simulink model "ProjectOverview"  (R2016a)
settings: Solver=VariableStepAuto  StartTime=0.0  StopTime=1  RelTol=1e-3
libraries: fl_lib x36, elec_lib x17, nesl_utility x6
settings Model: Creator=Peter  LastModifiedBy=Peter

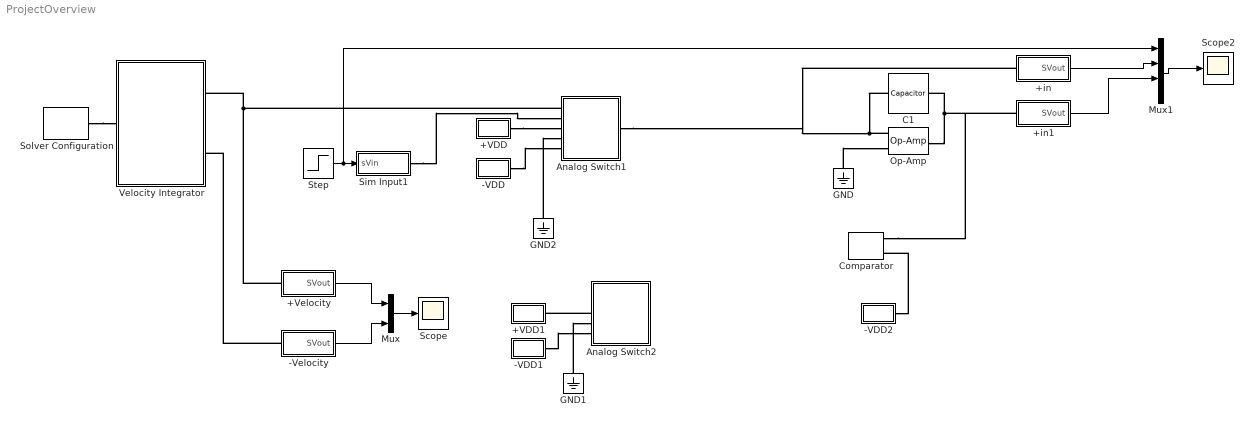
== system ProjectOverview ==
  +VDD : Subsystem
  +VDD1 : Subsystem
  +Velocity : Subsystem
  +in : Subsystem
  +in1 : Subsystem
  -VDD : Subsystem
  -VDD1 : Subsystem
  -VDD2 : Subsystem
  -Velocity : Subsystem
  Analog Switch1 : Subsystem
  Analog Switch2 : Subsystem
  C1 : fl_lib/Electrical/Electrical Elements/Capacitor  c=1e-6 F  r=1e-6 Ohm  g=0 1/Ohm  i_specify=off  i_priority=None  i=0 A  v_specify=off  v_priority=None  v=0 V  vc_specify=off  vc_priority=High  vc=0 V
  Comparator : elec_lib/Integrated Circuits/Comparator  V_OS=5 mV  V_OL=-14.3 V  V_OH=14.3 V  C_IN=0 pF  R_OUT=50 Ohm  Delay=0 s
  GND : fl_lib/Electrical/Electrical Elements/Electrical Reference
  GND1 : fl_lib/Electrical/Electrical Elements/Electrical Reference
  GND2 : fl_lib/Electrical/Electrical Elements/Electrical Reference
  Mux : Mux  Inputs=2
  Mux1 : Mux
  Op-Amp : fl_lib/Electrical/Electrical Elements/Op-Amp  outI_specify=off  outI_priority=None  outI=0 A
  Scope : Scope
  Scope2 : Scope
  Sim Input1 : Subsystem
  Solver Configuration : nesl_utility/Solver Configuration  PhysicalDomain=network_engine_domain  SubClassName=solver  LeftPortType=input  RightPortType=generic  Accelerate=off  Tones=[]  Harmonics=[]  SimulateNoise=off  Profile=off  UseLocalSampling=off  EnableSwitchedLinearOptims=on  FrequencyDomain=off  UseCCode=off  RelTol=0.001  AbsTol=1e-06  MinStep=1e-09  ToWorkspace=off  RevertToSquareIcSolve=off  NumHomotopyIterations=100  PhasorMode=off  PhasorModeNumHarmonics=1  OverrideAbsTol=off  DoDC=off  ResidualTolerance=1e-09  UseLocalSolver=off  LocalSolverChoice=NE_BACKWARD_EULER_ADVANCER  LocalSolverSampleTime=0.001  DoFixedCost=off  MaxNonlinIter=3  MaxModeIter=2  LinearAlgebra=Sparse  DelaysMemoryBudget=1024  AutomaticFiltering=on  FilteringTimeConstant=0.001
  Step : Step  Time=.5  Before=-10  After=10  SampleTime=0
  Velocity Integrator : Subsystem
  wires:
  +Velocity/1(SVout) -> Mux/1
  -Velocity/1(SVout) -> Mux/2
  Mux/1 -> Scope/1
  Mux1/1 -> Scope2/1
  +in/1(SVout) -> Mux1/2
  +in1/1(SVout) -> Mux1/3
  Step/1 -> Mux1/1, Sim Input1/1(sVin)
  connections:
  Solver Configuration/RConn1 -- Velocity Integrator/LConn1
  GND/LConn1 -- Op-Amp/LConn1
  Op-Amp/RConn1 -- Comparator/LConn2 -- +in1/LConn1 -- C1/RConn1
  +Velocity/LConn1 -- Analog Switch1/LConn1 -- Velocity Integrator/RConn1
  -Velocity/LConn1 -- Velocity Integrator/RConn2
  Op-Amp/LConn2 -- Analog Switch1/RConn1 -- +in/LConn1 -- C1/LConn1
  +VDD/RConn1 -- Analog Switch1/LConn3
  -VDD/RConn1 -- Analog Switch1/LConn5
  GND2/LConn1 -- Analog Switch1/LConn4
  Sim Input1/RConn1 -- Analog Switch1/LConn2
  Analog Switch2/LConn3 -- +VDD1/RConn1
  -VDD1/RConn1 -- Analog Switch2/LConn5
  GND1/LConn1 -- Analog Switch2/LConn4
  -VDD2/RConn1 -- Comparator/LConn1

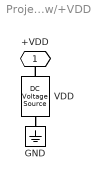
== system ProjectOverview/+VDD ==
  GND : fl_lib/Electrical/Electrical Elements/Electrical Reference
  VDD : fl_lib/Electrical/Electrical Sources/DC Voltage Source  v0=14.3 V
  +VDD : PMIOPort  Port=1  Side=Right
  connections:
  VDD/LConn1 -- +VDD/RConn1
  VDD/RConn1 -- GND/LConn1

== system ProjectOverview/+VDD1 ==
  GND : fl_lib/Electrical/Electrical Elements/Electrical Reference
  VDD : fl_lib/Electrical/Electrical Sources/DC Voltage Source  v0=14.3 V
  +VDD : PMIOPort  Port=1  Side=Right
  connections:
  VDD/LConn1 -- +VDD/RConn1
  VDD/RConn1 -- GND/LConn1

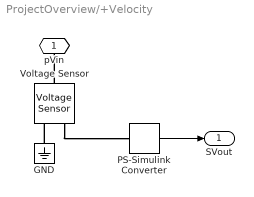
== system ProjectOverview/+Velocity ==
  GND : fl_lib/Electrical/Electrical Elements/Electrical Reference
  PS-Simulink Converter : nesl_utility/PS-Simulink Converter  PhysicalDomain=network_engine_domain  SubClassName=ps_output  LeftPortType=input  RightPortType=output  PseudoPeriodic=off  Frequencies=[]  Unit=V  AffineConversion=off
  Voltage Sensor : fl_lib/Electrical/Electrical Sensors/Voltage Sensor
  pVin : PMIOPort  Port=1  Side=Left
  SVout : Outport
  wires:
  PS-Simulink Converter/1 -> SVout/1
  connections:
  GND/LConn1 -- Voltage Sensor/RConn2
  Voltage Sensor/LConn1 -- pVin/RConn1
  Voltage Sensor/RConn1 -- PS-Simulink Converter/LConn1

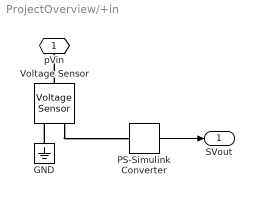
== system ProjectOverview/+in ==
  GND : fl_lib/Electrical/Electrical Elements/Electrical Reference
  PS-Simulink Converter : nesl_utility/PS-Simulink Converter  PhysicalDomain=network_engine_domain  SubClassName=ps_output  LeftPortType=input  RightPortType=output  PseudoPeriodic=off  Frequencies=[]  Unit=V  AffineConversion=off
  Voltage Sensor : fl_lib/Electrical/Electrical Sensors/Voltage Sensor
  pVin : PMIOPort  Port=1  Side=Left
  SVout : Outport
  wires:
  PS-Simulink Converter/1 -> SVout/1
  connections:
  GND/LConn1 -- Voltage Sensor/RConn2
  Voltage Sensor/LConn1 -- pVin/RConn1
  Voltage Sensor/RConn1 -- PS-Simulink Converter/LConn1

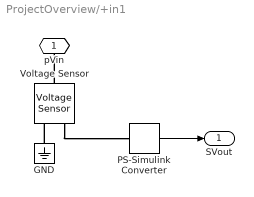
== system ProjectOverview/+in1 ==
  GND : fl_lib/Electrical/Electrical Elements/Electrical Reference
  PS-Simulink Converter : nesl_utility/PS-Simulink Converter  PhysicalDomain=network_engine_domain  SubClassName=ps_output  LeftPortType=input  RightPortType=output  PseudoPeriodic=off  Frequencies=[]  Unit=V  AffineConversion=off
  Voltage Sensor : fl_lib/Electrical/Electrical Sensors/Voltage Sensor
  pVin : PMIOPort  Port=1  Side=Left
  SVout : Outport
  wires:
  PS-Simulink Converter/1 -> SVout/1
  connections:
  GND/LConn1 -- Voltage Sensor/RConn2
  Voltage Sensor/LConn1 -- pVin/RConn1
  Voltage Sensor/RConn1 -- PS-Simulink Converter/LConn1

== system ProjectOverview/-VDD ==
  GND : fl_lib/Electrical/Electrical Elements/Electrical Reference
  VDD : fl_lib/Electrical/Electrical Sources/DC Voltage Source  v0=14.3 V
  -VDD : PMIOPort  Port=1  Side=Right
  connections:
  VDD/RConn1 -- -VDD/RConn1
  GND/LConn1 -- VDD/LConn1

== system ProjectOverview/-VDD1 ==
  GND : fl_lib/Electrical/Electrical Elements/Electrical Reference
  VDD : fl_lib/Electrical/Electrical Sources/DC Voltage Source  v0=14.3 V
  -VDD : PMIOPort  Port=1  Side=Right
  connections:
  VDD/RConn1 -- -VDD/RConn1
  GND/LConn1 -- VDD/LConn1

== system ProjectOverview/-VDD2 ==
  GND : fl_lib/Electrical/Electrical Elements/Electrical Reference
  VDD : fl_lib/Electrical/Electrical Sources/DC Voltage Source  v0=14.3 V
  -VDD : PMIOPort  Port=1  Side=Right
  connections:
  VDD/RConn1 -- -VDD/RConn1
  GND/LConn1 -- VDD/LConn1

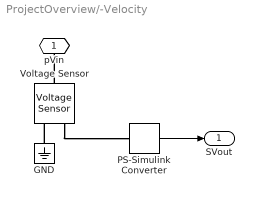
== system ProjectOverview/-Velocity ==
  GND : fl_lib/Electrical/Electrical Elements/Electrical Reference
  PS-Simulink Converter : nesl_utility/PS-Simulink Converter  PhysicalDomain=network_engine_domain  SubClassName=ps_output  LeftPortType=input  RightPortType=output  PseudoPeriodic=off  Frequencies=[]  Unit=V  AffineConversion=off
  Voltage Sensor : fl_lib/Electrical/Electrical Sensors/Voltage Sensor
  pVin : PMIOPort  Port=1  Side=Left
  SVout : Outport
  wires:
  PS-Simulink Converter/1 -> SVout/1
  connections:
  GND/LConn1 -- Voltage Sensor/RConn2
  Voltage Sensor/LConn1 -- pVin/RConn1
  Voltage Sensor/RConn1 -- PS-Simulink Converter/LConn1

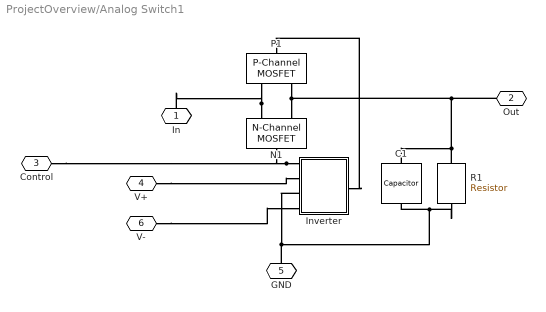
== system ProjectOverview/Analog Switch1 ==
  C1 : fl_lib/Electrical/Electrical Elements/Capacitor  c=1e-6 F  r=1e-6 Ohm  g=0 1/Ohm  i_specify=off  i_priority=None  i=0 A  v_specify=off  v_priority=None  v=0 V  vc_specify=off  vc_priority=High  vc=0 V
  Inverter : Subsystem
  N1 : elec_lib/Semiconductor Devices/N-Channel MOSFET  parameterization=1  prmDatasheet=1  prmEquCoeff=1  Beta=5 A/V^2  Rds=0.025 Ohm  Id=6 A  Vgs=10 V  Vth=1.7 V  lam=0 1/V  Tmeas=25 degC  RS=1e-4 Ohm  RD=0.01 Ohm  C_param=1  C_GS=270 pF  C_GD=80 pF  C_DS=0 pF  C_iss=350 pF  C_rss=80 pF  C_oss=0 pF  C_GS_vec=[ 270 300 290 280 295 255 ] pF  C_GD_vec=[ 450 400 300 190 95 55 ] pF  C_DS_vec=[ 450 410 390 230 175 115 ] pF  C_iss_vec=[ 720 700 590 470 390 310 ] pF  C_rss_vec=[ 450 400 300 190 95 55 ] pF  C_oss_vec=[ 900 810 690 420 270 170 ] pF  C_Vds_vec=[ 0.1 0.3 1 3 10 30 ] V  charge_linearity_param=1  C_OX=200 pF  V_C_OX=-0.5 V  dVth_dT=-6 mV/K  Rds_T2=0.037 Ohm  Tmeas2=125 degC  BEXDatasheet=-1.5  BEXEquCoeff=-1.5  TdeviceDatasheet=25 degC  TdeviceEquCoeff=25 degC  Rth=[ 0 10 ] K/W  thermal_mass_parameterization=1  thermal_mass=[ 0 1 ] J/K  thermal_time_constant=[ 0 10 ] s  thermal_mass_initial_temperatures=[ 25 25 ] degC
  P1 : elec_lib/Semiconductor Devices/P-Channel MOSFET  parameterization=1  prmDatasheet=1  prmEquCoeff=1  Beta=2 A/V^2  Rds=0.167 Ohm  Id=-2.5 A  Vgs=-4.5 V  Vth=-1.4 V  lam=0 1/V  Tmeas=25 degC  RS=1e-4 Ohm  RD=0.01 Ohm  C_param=1  C_GS=158 pF  C_GD=24 pF  C_DS=0 pF  C_iss=182 pF  C_rss=24 pF  C_oss=0 pF  C_GS_vec=[ 150 150 150 150 150 150 ] pF  C_GD_vec=[ 75 60 50 35 25 20 ] pF  C_DS_vec=[ 105 100 75 45 35 25 ] pF  C_iss_vec=[ 225 210 200 185 175 170 ] pF  C_rss_vec=[ 75 60 50 35 25 20 ] pF  C_oss_vec=[ 180 160 125 80 60 45 ] pF  C_Vsd_vec=[ 0.1 0.3 1 3 10 30 ] V  charge_linearity_param=1  C_OX=200 pF  V_C_OX=0.5 V  dVth_dT=2 mV/K  Rds_T2=0.25 Ohm  Tmeas2=125 degC  BEXDatasheet=-1.5  BEXEquCoeff=-1.5  TdeviceDatasheet=25 degC  TdeviceEquCoeff=25 degC  Rth=[ 0 10 ] K/W  thermal_mass_parameterization=1  thermal_mass=[ 0 1 ] J/K  thermal_time_constant=[ 0 10 ] s  thermal_mass_initial_temperatures=[ 25 25 ] degC
  R1 : elec_lib/Passive Devices/Resistor  R=100e3 Ohm  R_tol=5  enable_R_tol=0  tol_distribution=1  nSigma=4  enable_operating_limits=0  operating_limit_action=2  max_working_voltage=100 V  power_rating=1 W  enable_faults=0  fault_action=1  R_faulted=Inf Ohm  enable_temporal_fault=0  t_fault=1 s  enable_behavioral_fault=0  max_permissible_current=1 A  t_fail_on_current=1 s  noise_mode=0  sample_time=0.001 s  repeatability=1  auto_seed=1099607551  user_seed=0  Tdevice=25 degC  alpha=0.00393 1/K  Tmeas=25 degC  thermal_mass=100 J/K  initial_temperature=25 degC  power_derating_T1=70 degC  power_derating_T2=155 degC  operating_temperature_range_vec=[ -50 150 ] degC
  In : PMIOPort  Port=1  Side=Left
  Out : PMIOPort  Port=2  Side=Right
  Control : PMIOPort  Port=3  Side=Left
  V+ : PMIOPort  Port=4  Side=Left
  GND : PMIOPort  Port=5  Side=Left
  V- : PMIOPort  Port=6  Side=Left
  connections:
  GND/RConn1 -- C1/RConn1 -- R1/RConn1 -- Inverter/LConn3
  Inverter/RConn1 -- P1/LConn1
  Inverter/LConn1 -- N1/LConn1 -- Control/RConn1
  C1/LConn1 -- R1/LConn1 -- N1/RConn1 -- P1/RConn2 -- Out/RConn1
  N1/RConn2 -- P1/RConn1 -- In/RConn1
  V+/RConn1 -- Inverter/LConn2
  V-/RConn1 -- Inverter/LConn4

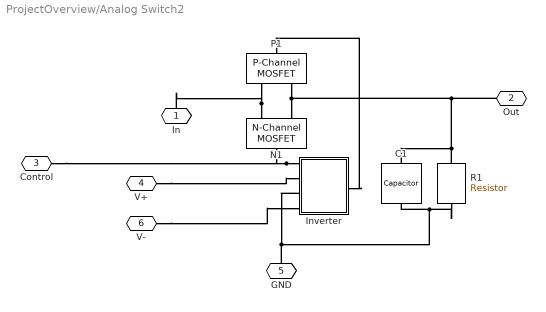
== system ProjectOverview/Analog Switch2 ==
  C1 : fl_lib/Electrical/Electrical Elements/Capacitor  c=1e-6 F  r=1e-6 Ohm  g=0 1/Ohm  i_specify=off  i_priority=None  i=0 A  v_specify=off  v_priority=None  v=0 V  vc_specify=off  vc_priority=High  vc=0 V
  Inverter : Subsystem
  N1 : elec_lib/Semiconductor Devices/N-Channel MOSFET  parameterization=1  prmDatasheet=1  prmEquCoeff=1  Beta=5 A/V^2  Rds=0.025 Ohm  Id=6 A  Vgs=10 V  Vth=1.7 V  lam=0 1/V  Tmeas=25 degC  RS=1e-4 Ohm  RD=0.01 Ohm  C_param=1  C_GS=270 pF  C_GD=80 pF  C_DS=0 pF  C_iss=350 pF  C_rss=80 pF  C_oss=0 pF  C_GS_vec=[ 270 300 290 280 295 255 ] pF  C_GD_vec=[ 450 400 300 190 95 55 ] pF  C_DS_vec=[ 450 410 390 230 175 115 ] pF  C_iss_vec=[ 720 700 590 470 390 310 ] pF  C_rss_vec=[ 450 400 300 190 95 55 ] pF  C_oss_vec=[ 900 810 690 420 270 170 ] pF  C_Vds_vec=[ 0.1 0.3 1 3 10 30 ] V  charge_linearity_param=1  C_OX=200 pF  V_C_OX=-0.5 V  dVth_dT=-6 mV/K  Rds_T2=0.037 Ohm  Tmeas2=125 degC  BEXDatasheet=-1.5  BEXEquCoeff=-1.5  TdeviceDatasheet=25 degC  TdeviceEquCoeff=25 degC  Rth=[ 0 10 ] K/W  thermal_mass_parameterization=1  thermal_mass=[ 0 1 ] J/K  thermal_time_constant=[ 0 10 ] s  thermal_mass_initial_temperatures=[ 25 25 ] degC
  P1 : elec_lib/Semiconductor Devices/P-Channel MOSFET  parameterization=1  prmDatasheet=1  prmEquCoeff=1  Beta=2 A/V^2  Rds=0.167 Ohm  Id=-2.5 A  Vgs=-4.5 V  Vth=-1.4 V  lam=0 1/V  Tmeas=25 degC  RS=1e-4 Ohm  RD=0.01 Ohm  C_param=1  C_GS=158 pF  C_GD=24 pF  C_DS=0 pF  C_iss=182 pF  C_rss=24 pF  C_oss=0 pF  C_GS_vec=[ 150 150 150 150 150 150 ] pF  C_GD_vec=[ 75 60 50 35 25 20 ] pF  C_DS_vec=[ 105 100 75 45 35 25 ] pF  C_iss_vec=[ 225 210 200 185 175 170 ] pF  C_rss_vec=[ 75 60 50 35 25 20 ] pF  C_oss_vec=[ 180 160 125 80 60 45 ] pF  C_Vsd_vec=[ 0.1 0.3 1 3 10 30 ] V  charge_linearity_param=1  C_OX=200 pF  V_C_OX=0.5 V  dVth_dT=2 mV/K  Rds_T2=0.25 Ohm  Tmeas2=125 degC  BEXDatasheet=-1.5  BEXEquCoeff=-1.5  TdeviceDatasheet=25 degC  TdeviceEquCoeff=25 degC  Rth=[ 0 10 ] K/W  thermal_mass_parameterization=1  thermal_mass=[ 0 1 ] J/K  thermal_time_constant=[ 0 10 ] s  thermal_mass_initial_temperatures=[ 25 25 ] degC
  R1 : elec_lib/Passive Devices/Resistor  R=100e3 Ohm  R_tol=5  enable_R_tol=0  tol_distribution=1  nSigma=4  enable_operating_limits=0  operating_limit_action=2  max_working_voltage=100 V  power_rating=1 W  enable_faults=0  fault_action=1  R_faulted=Inf Ohm  enable_temporal_fault=0  t_fault=1 s  enable_behavioral_fault=0  max_permissible_current=1 A  t_fail_on_current=1 s  noise_mode=0  sample_time=0.001 s  repeatability=1  auto_seed=2017132988  user_seed=0  Tdevice=25 degC  alpha=0.00393 1/K  Tmeas=25 degC  thermal_mass=100 J/K  initial_temperature=25 degC  power_derating_T1=70 degC  power_derating_T2=155 degC  operating_temperature_range_vec=[ -50 150 ] degC
  In : PMIOPort  Port=1  Side=Left
  Out : PMIOPort  Port=2  Side=Right
  Control : PMIOPort  Port=3  Side=Left
  V+ : PMIOPort  Port=4  Side=Left
  GND : PMIOPort  Port=5  Side=Left
  V- : PMIOPort  Port=6  Side=Left
  connections:
  GND/RConn1 -- C1/RConn1 -- R1/RConn1 -- Inverter/LConn3
  Inverter/RConn1 -- P1/LConn1
  Inverter/LConn1 -- N1/LConn1 -- Control/RConn1
  C1/LConn1 -- R1/LConn1 -- N1/RConn1 -- P1/RConn2 -- Out/RConn1
  N1/RConn2 -- P1/RConn1 -- In/RConn1
  V+/RConn1 -- Inverter/LConn2
  V-/RConn1 -- Inverter/LConn4

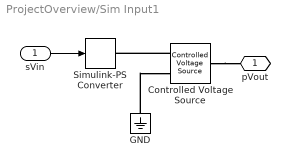
== system ProjectOverview/Sim Input1 ==
  sVin : Inport
  Controlled Voltage Source : fl_lib/Electrical/Electrical Sources/Controlled Voltage Source
  GND : fl_lib/Electrical/Electrical Elements/Electrical Reference
  Simulink-PS Converter : nesl_utility/Simulink-PS Converter  PhysicalDomain=network_engine_domain  SubClassName=ps_input  LeftPortType=input  RightPortType=output  PseudoPeriodic=off  Frequencies=[]  NoiseDistribution=none  NoiseParameters=[]  Unit=V  AffineConversion=off  InputFiltering=off  SimscapeFilterOrder=1  InputFilterTimeConstant=0.001  UdotUserProvided=1
  pVout : PMIOPort  Port=1  Side=Right
  wires:
  sVin/1 -> Simulink-PS Converter/1
  connections:
  Controlled Voltage Source/RConn1 -- Simulink-PS Converter/RConn1
  GND/LConn1 -- Controlled Voltage Source/RConn2
  Controlled Voltage Source/LConn1 -- pVout/RConn1

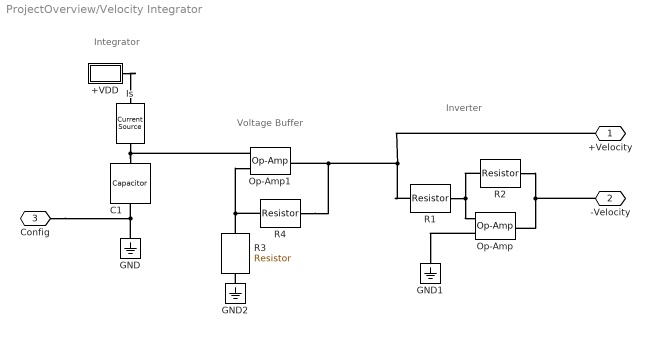
== system ProjectOverview/Velocity Integrator ==
  note: Inverter
  note: Voltage Buffer
  note: Integrator
  +VDD : Subsystem
  C1 : elec_lib/Passive Devices/Capacitor  enable_table=0  c=100e-6 F  Cvec=[ 1e-5 1e-6 ] F  Vvec=[ 0 10 ] V  CV_table_symmetry=1  C_tol=5  enable_C_tol=0  tol_distribution=1  nSigma=4  r=1e-6 Ohm  g=0 1/Ohm  initV=0 V  enable_operating_limits=0  operating_limit_action=2  max_working_voltage_range=[ -25 25 ] V  power_rating=1 W  enable_faults=0  fault_action=1  Cscale_faulted=100  R_faulted=0.001 Ohm  G_faulted=0 1/Ohm  tau_fault=0.001 s  enable_temporal_fault=0  t_fault=1 s  enable_behavioral_fault=0  max_permissible_voltage_range=[ -100 100 ] V  t_fail_on_voltage=1 s
  GND : fl_lib/Electrical/Electrical Elements/Electrical Reference
  GND1 : fl_lib/Electrical/Electrical Elements/Electrical Reference
  GND2 : fl_lib/Electrical/Electrical Elements/Electrical Reference
  Is : elec_lib/Sources/Current Source  dc_current=1.4/220e3 A  ac_current=0 A  ac_shift=0 deg  ac_frequency=60 Hz  noise_mode=0  PSD=0 A^2/Hz  sample_time=0.001 s  repeatability=1  auto_seed=326277333  user_seed=0
  Op-Amp : fl_lib/Electrical/Electrical Elements/Op-Amp  outI_specify=off  outI_priority=None  outI=0 A
  Op-Amp1 : fl_lib/Electrical/Electrical Elements/Op-Amp  outI_specify=off  outI_priority=None  outI=0 A
  R1 : elec_lib/Passive Devices/Resistor  R=200e3 Ohm  R_tol=5  enable_R_tol=0  tol_distribution=1  nSigma=4  enable_operating_limits=0  operating_limit_action=2  max_working_voltage=100 V  power_rating=1 W  enable_faults=0  fault_action=1  R_faulted=Inf Ohm  enable_temporal_fault=0  t_fault=1 s  enable_behavioral_fault=0  max_permissible_current=1 A  t_fail_on_current=1 s  noise_mode=0  sample_time=0.001 s  repeatability=1  auto_seed=1671295314  user_seed=0  Tdevice=25 degC  alpha=0.00393 1/K  Tmeas=25 degC  thermal_mass=100 J/K  initial_temperature=25 degC  power_derating_T1=70 degC  power_derating_T2=155 degC  operating_temperature_range_vec=[ -50 150 ] degC
  R2 : elec_lib/Passive Devices/Resistor  R=200e3 Ohm  R_tol=5  enable_R_tol=0  tol_distribution=1  nSigma=4  enable_operating_limits=0  operating_limit_action=2  max_working_voltage=100 V  power_rating=1 W  enable_faults=0  fault_action=1  R_faulted=Inf Ohm  enable_temporal_fault=0  t_fault=1 s  enable_behavioral_fault=0  max_permissible_current=1 A  t_fail_on_current=1 s  noise_mode=0  sample_time=0.001 s  repeatability=1  auto_seed=253534306  user_seed=0  Tdevice=25 degC  alpha=0.00393 1/K  Tmeas=25 degC  thermal_mass=100 J/K  initial_temperature=25 degC  power_derating_T1=70 degC  power_derating_T2=155 degC  operating_temperature_range_vec=[ -50 150 ] degC
  R3 : elec_lib/Passive Devices/Resistor  R=200e3 Ohm  R_tol=5  enable_R_tol=0  tol_distribution=1  nSigma=4  enable_operating_limits=0  operating_limit_action=2  max_working_voltage=100 V  power_rating=1 W  enable_faults=0  fault_action=1  R_faulted=Inf Ohm  enable_temporal_fault=0  t_fault=1 s  enable_behavioral_fault=0  max_permissible_current=1 A  t_fail_on_current=1 s  noise_mode=0  sample_time=0.001 s  repeatability=1  auto_seed=357839259  user_seed=0  Tdevice=25 degC  alpha=0.00393 1/K  Tmeas=25 degC  thermal_mass=100 J/K  initial_temperature=25 degC  power_derating_T1=70 degC  power_derating_T2=155 degC  operating_temperature_range_vec=[ -50 150 ] degC
  R4 : elec_lib/Passive Devices/Resistor  R=200e3 Ohm  R_tol=5  enable_R_tol=0  tol_distribution=1  nSigma=4  enable_operating_limits=0  operating_limit_action=2  max_working_voltage=100 V  power_rating=1 W  enable_faults=0  fault_action=1  R_faulted=Inf Ohm  enable_temporal_fault=0  t_fault=1 s  enable_behavioral_fault=0  max_permissible_current=1 A  t_fail_on_current=1 s  noise_mode=0  sample_time=0.001 s  repeatability=1  auto_seed=2195185148  user_seed=0  Tdevice=25 degC  alpha=0.00393 1/K  Tmeas=25 degC  thermal_mass=100 J/K  initial_temperature=25 degC  power_derating_T1=70 degC  power_derating_T2=155 degC  operating_temperature_range_vec=[ -50 150 ] degC
  +Velocity : PMIOPort  Port=1  Side=Right
  -Velocity : PMIOPort  Port=2  Side=Right
  Config : PMIOPort  Port=3  Side=Left
  connections:
  +VDD/RConn1 -- Is/RConn1
  GND2/LConn1 -- R3/RConn1
  Is/LConn1 -- C1/LConn1 -- Op-Amp1/LConn1
  GND/LConn1 -- Config/RConn1 -- C1/RConn1
  R1/RConn1 -- R2/LConn1 -- Op-Amp/LConn2
  R3/LConn1 -- R4/LConn1 -- Op-Amp1/LConn2
  R2/RConn1 -- -Velocity/RConn1 -- Op-Amp/RConn1
  Op-Amp/LConn1 -- GND1/LConn1
  R4/RConn1 -- +Velocity/RConn1 -- R1/LConn1 -- Op-Amp1/RConn1

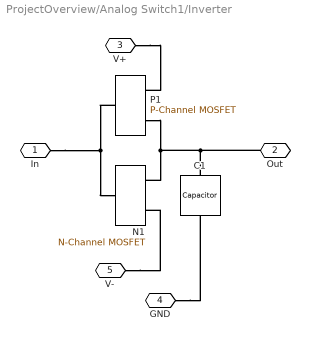
== system ProjectOverview/Analog Switch1/Inverter ==
  C1 : fl_lib/Electrical/Electrical Elements/Capacitor  c=1e-6 F  r=1e-6 Ohm  g=0 1/Ohm  i_specify=off  i_priority=None  i=0 A  v_specify=off  v_priority=None  v=0 V  vc_specify=off  vc_priority=High  vc=0 V
  N1 : elec_lib/Semiconductor Devices/N-Channel MOSFET  parameterization=1  prmDatasheet=1  prmEquCoeff=1  Beta=5 A/V^2  Rds=0.025 Ohm  Id=6 A  Vgs=10 V  Vth=1.7 V  lam=0 1/V  Tmeas=25 degC  RS=1e-4 Ohm  RD=0.01 Ohm  C_param=1  C_GS=270 pF  C_GD=80 pF  C_DS=0 pF  C_iss=350 pF  C_rss=80 pF  C_oss=0 pF  C_GS_vec=[ 270 300 290 280 295 255 ] pF  C_GD_vec=[ 450 400 300 190 95 55 ] pF  C_DS_vec=[ 450 410 390 230 175 115 ] pF  C_iss_vec=[ 720 700 590 470 390 310 ] pF  C_rss_vec=[ 450 400 300 190 95 55 ] pF  C_oss_vec=[ 900 810 690 420 270 170 ] pF  C_Vds_vec=[ 0.1 0.3 1 3 10 30 ] V  charge_linearity_param=1  C_OX=200 pF  V_C_OX=-0.5 V  dVth_dT=-6 mV/K  Rds_T2=0.037 Ohm  Tmeas2=125 degC  BEXDatasheet=-1.5  BEXEquCoeff=-1.5  TdeviceDatasheet=25 degC  TdeviceEquCoeff=25 degC  Rth=[ 0 10 ] K/W  thermal_mass_parameterization=1  thermal_mass=[ 0 1 ] J/K  thermal_time_constant=[ 0 10 ] s  thermal_mass_initial_temperatures=[ 25 25 ] degC
  P1 : elec_lib/Semiconductor Devices/P-Channel MOSFET  parameterization=1  prmDatasheet=1  prmEquCoeff=1  Beta=2 A/V^2  Rds=0.167 Ohm  Id=-2.5 A  Vgs=-4.5 V  Vth=-1.4 V  lam=0 1/V  Tmeas=25 degC  RS=1e-4 Ohm  RD=0.01 Ohm  C_param=1  C_GS=158 pF  C_GD=24 pF  C_DS=0 pF  C_iss=182 pF  C_rss=24 pF  C_oss=0 pF  C_GS_vec=[ 150 150 150 150 150 150 ] pF  C_GD_vec=[ 75 60 50 35 25 20 ] pF  C_DS_vec=[ 105 100 75 45 35 25 ] pF  C_iss_vec=[ 225 210 200 185 175 170 ] pF  C_rss_vec=[ 75 60 50 35 25 20 ] pF  C_oss_vec=[ 180 160 125 80 60 45 ] pF  C_Vsd_vec=[ 0.1 0.3 1 3 10 30 ] V  charge_linearity_param=1  C_OX=200 pF  V_C_OX=0.5 V  dVth_dT=2 mV/K  Rds_T2=0.25 Ohm  Tmeas2=125 degC  BEXDatasheet=-1.5  BEXEquCoeff=-1.5  TdeviceDatasheet=25 degC  TdeviceEquCoeff=25 degC  Rth=[ 0 10 ] K/W  thermal_mass_parameterization=1  thermal_mass=[ 0 1 ] J/K  thermal_time_constant=[ 0 10 ] s  thermal_mass_initial_temperatures=[ 25 25 ] degC
  In : PMIOPort  Port=1  Side=Left
  Out : PMIOPort  Port=2  Side=Right
  V+ : PMIOPort  Port=3  Side=Left
  GND : PMIOPort  Port=4  Side=Left
  V- : PMIOPort  Port=5  Side=Left
  connections:
  P1/LConn1 -- N1/LConn1 -- In/RConn1
  C1/LConn1 -- N1/RConn1 -- P1/RConn2 -- Out/RConn1
  V+/RConn1 -- P1/RConn1
  V-/RConn1 -- N1/RConn2
  GND/RConn1 -- C1/RConn1

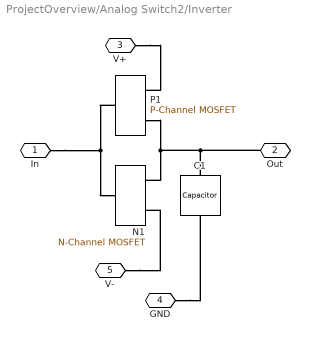
== system ProjectOverview/Analog Switch2/Inverter ==
  C1 : fl_lib/Electrical/Electrical Elements/Capacitor  c=1e-6 F  r=1e-6 Ohm  g=0 1/Ohm  i_specify=off  i_priority=None  i=0 A  v_specify=off  v_priority=None  v=0 V  vc_specify=off  vc_priority=High  vc=0 V
  N1 : elec_lib/Semiconductor Devices/N-Channel MOSFET  parameterization=1  prmDatasheet=1  prmEquCoeff=1  Beta=5 A/V^2  Rds=0.025 Ohm  Id=6 A  Vgs=10 V  Vth=1.7 V  lam=0 1/V  Tmeas=25 degC  RS=1e-4 Ohm  RD=0.01 Ohm  C_param=1  C_GS=270 pF  C_GD=80 pF  C_DS=0 pF  C_iss=350 pF  C_rss=80 pF  C_oss=0 pF  C_GS_vec=[ 270 300 290 280 295 255 ] pF  C_GD_vec=[ 450 400 300 190 95 55 ] pF  C_DS_vec=[ 450 410 390 230 175 115 ] pF  C_iss_vec=[ 720 700 590 470 390 310 ] pF  C_rss_vec=[ 450 400 300 190 95 55 ] pF  C_oss_vec=[ 900 810 690 420 270 170 ] pF  C_Vds_vec=[ 0.1 0.3 1 3 10 30 ] V  charge_linearity_param=1  C_OX=200 pF  V_C_OX=-0.5 V  dVth_dT=-6 mV/K  Rds_T2=0.037 Ohm  Tmeas2=125 degC  BEXDatasheet=-1.5  BEXEquCoeff=-1.5  TdeviceDatasheet=25 degC  TdeviceEquCoeff=25 degC  Rth=[ 0 10 ] K/W  thermal_mass_parameterization=1  thermal_mass=[ 0 1 ] J/K  thermal_time_constant=[ 0 10 ] s  thermal_mass_initial_temperatures=[ 25 25 ] degC
  P1 : elec_lib/Semiconductor Devices/P-Channel MOSFET  parameterization=1  prmDatasheet=1  prmEquCoeff=1  Beta=2 A/V^2  Rds=0.167 Ohm  Id=-2.5 A  Vgs=-4.5 V  Vth=-1.4 V  lam=0 1/V  Tmeas=25 degC  RS=1e-4 Ohm  RD=0.01 Ohm  C_param=1  C_GS=158 pF  C_GD=24 pF  C_DS=0 pF  C_iss=182 pF  C_rss=24 pF  C_oss=0 pF  C_GS_vec=[ 150 150 150 150 150 150 ] pF  C_GD_vec=[ 75 60 50 35 25 20 ] pF  C_DS_vec=[ 105 100 75 45 35 25 ] pF  C_iss_vec=[ 225 210 200 185 175 170 ] pF  C_rss_vec=[ 75 60 50 35 25 20 ] pF  C_oss_vec=[ 180 160 125 80 60 45 ] pF  C_Vsd_vec=[ 0.1 0.3 1 3 10 30 ] V  charge_linearity_param=1  C_OX=200 pF  V_C_OX=0.5 V  dVth_dT=2 mV/K  Rds_T2=0.25 Ohm  Tmeas2=125 degC  BEXDatasheet=-1.5  BEXEquCoeff=-1.5  TdeviceDatasheet=25 degC  TdeviceEquCoeff=25 degC  Rth=[ 0 10 ] K/W  thermal_mass_parameterization=1  thermal_mass=[ 0 1 ] J/K  thermal_time_constant=[ 0 10 ] s  thermal_mass_initial_temperatures=[ 25 25 ] degC
  In : PMIOPort  Port=1  Side=Left
  Out : PMIOPort  Port=2  Side=Right
  V+ : PMIOPort  Port=3  Side=Left
  GND : PMIOPort  Port=4  Side=Left
  V- : PMIOPort  Port=5  Side=Left
  connections:
  P1/LConn1 -- N1/LConn1 -- In/RConn1
  C1/LConn1 -- N1/RConn1 -- P1/RConn2 -- Out/RConn1
  V+/RConn1 -- P1/RConn1
  V-/RConn1 -- N1/RConn2
  GND/RConn1 -- C1/RConn1

== system ProjectOverview/Velocity Integrator/+VDD ==
  GND : fl_lib/Electrical/Electrical Elements/Electrical Reference
  VDD : fl_lib/Electrical/Electrical Sources/DC Voltage Source  v0=14.3 V
  +VDD : PMIOPort  Port=1  Side=Right
  connections:
  VDD/LConn1 -- +VDD/RConn1
  VDD/RConn1 -- GND/LConn1
